simulink model "Modele_Principale"  (R2022b)
settings: Solver=ode3  StartTime=0.0  StopTime=150  FixedStep=0.05  RelTol=1e-3
model workspace (MAT data in the model file):
  D_Mesure = 0
values from neighbouring files (symbols this model uses):
  Acceleration_Max = 3.2    [Matlab_WorkSpace.mat]
  Distance_initial = 8    [Matlab_WorkSpace.mat]
  Frein_Max = -9    [Matlab_WorkSpace.mat]
  glissement = 0.22    [Matlab_WorkSpace.mat]
  r = 0.3    [Matlab_WorkSpace.mat]
  vehicule_half_length = 2.5    [Matlab_WorkSpace.mat]
libraries: sim3dautolib x2, slpidlib x2, sim3dprobsensorlib x1, sim3dlib x1
settings Model: Creator=Yoamiri  LastModifiedBy=Yoamiri
settings OptimizationCC: DefaultParameterBehavior=Inlined  EnhancedBackFolding=on  PassReuseOutputArgsAs=Individual arguments  ZeroExternalMemoryAtStartup=off  ZeroInternalMemoryAtStartup=off  OptimizeBlockOrder=speed  DifferentSizesBufferReuse=on  OptimizationCustomize=off  EfficientTunableParamExpr=on
settings DebuggingCC: ParameterTunabilityLossMsg=error
settings HardwareCC: ProdBitPerPointer=32  ProdBitPerSizeT=32  ProdBitPerPtrDiffT=32  ProdLargestAtomicFloat=None  ProdWordSize=32  ProdHWDeviceType=Atmel->AVR (32-bit)
settings SFSimCC: MATLABDynamicMemAlloc=off
settings RTWCC: Description=Embedded Coder  SystemTargetFile=ert.tlc  TemplateMakefile=ert_default_tmf  PortableWordSizes=on  CreateSILPILBlock=SIL
settings CodeAppCC: ForceParamTrailComments=on  IgnoreCustomStorageClasses=off  OperatorAnnotations=on  SimulinkDataObjDesc=on  SFDataObjDesc=on  InsertBlockDesc=on
settings ERTTargetCC: TargetLangStandard=C99 (ISO)  GenerateSampleERTMain=on  SupportVariableSizeSignals=on  InlinedParameterPlacement=NonHierarchical  ERTCustomFileTemplate=example_file_process.tlc

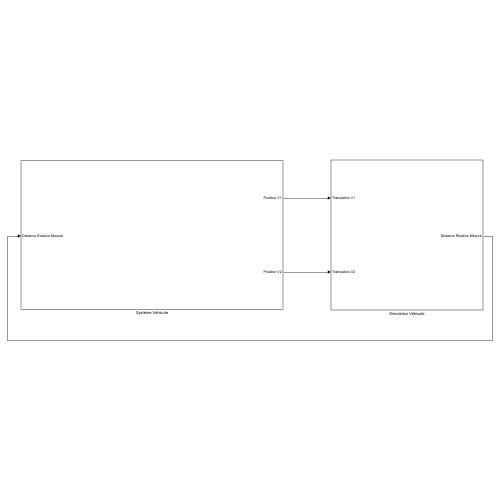
[thumbnail: Simulink's stored preview of the top-level diagram]
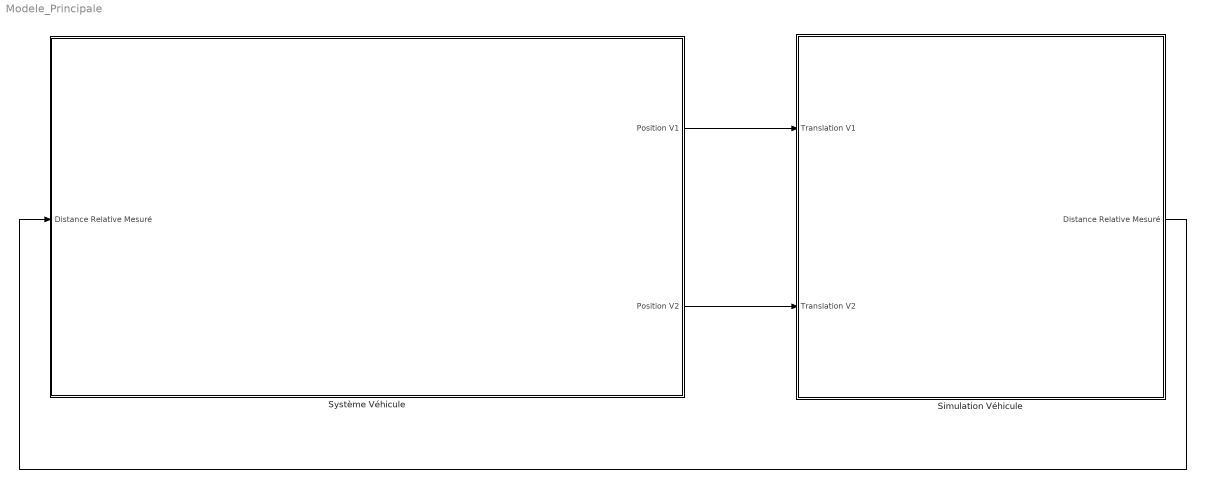
== system Modele_Principale ==
  Simulation Véhicule : Subsystem
  Système Véhicule : Subsystem
  wires:
  Système Véhicule/1(Position V1) -> Simulation Véhicule/1(Translation V1)
  Système Véhicule/2(Position V2) -> Simulation Véhicule/2(Translation V2)
  Simulation Véhicule/1(Distance Relative Mesuré) -> Système Véhicule/1(Distance Relative Mesuré)

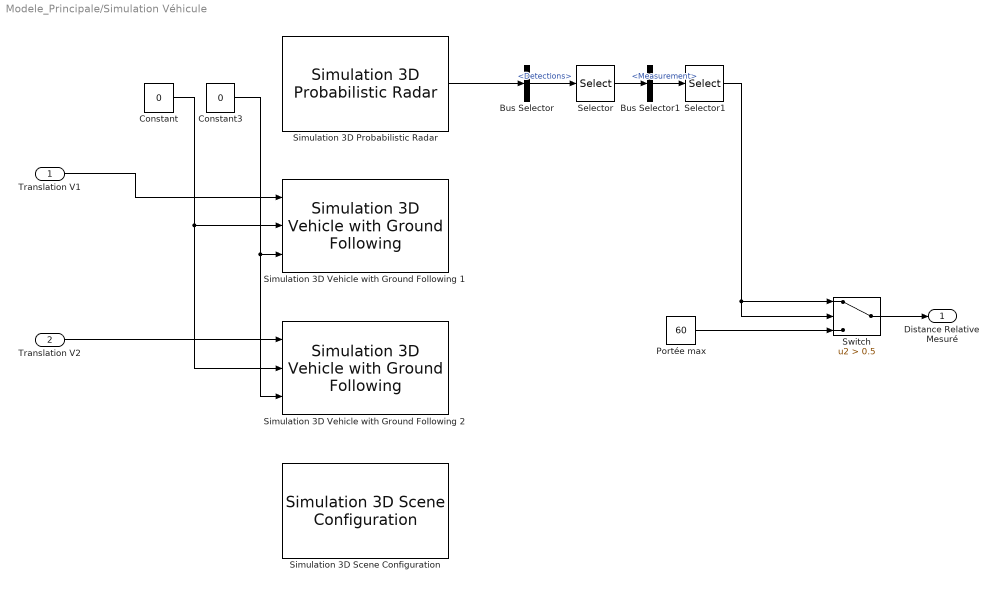
== system Modele_Principale/Simulation Véhicule ==
  Translation V1 : Inport
  Translation V2 : Inport  Port=2
  Bus Selector : BusSelector  OutputSignals=Detections
  Bus Selector1 : BusSelector  OutputSignals=Measurement
  Constant : Constant  Value=0
  Constant3 : Constant  Value=0
  Portée max : Constant  Value=60
  Selector : Selector  InputPortWidth=50  IndexOptions=Index vector (dialog)  Indices=[1]  OutputSizes=1
  Selector1 : Selector  InputPortWidth=6  IndexOptions=Index vector (dialog)  Indices=[1]  OutputSizes=1
  Simulation 3D Probabilistic Radar : sim3dprobsensorlib/Simulation 3D Probabilistic Radar  Priority=1  sensorTag=Sim3dSensor1  sensorId=1  sensorName=Sim3dSensor1  vehTagList={'Scene Origin';'Vehicule_Leader';'Vehicule_Suiveur'}  vehTag=Vehicule_Suiveur  mountLoc=Front bumper  offsetFlag=off  tmountOffset=[2.42, 0, 0.6]  rmountOffset=[0, 0, 0]  AzimuthResolution=4  ElevationResolution=10  RangeResolution=2.5  RangeRateResolution=0.5  AzimuthBiasFraction=0.1  ElevationBiasFraction=0.1  RangeBiasFraction=0.05  RangeRateBiasFraction=0.05  FieldOfView=[ 50, 10 ]  DetectionRange=[ 0.5, 200 ]  RangeRateLimits=[ -100, 100 ]  DetectionProbability=0.95  FalseAlarmRate=1e-6  ReferenceRange=180  ReferenceRCS=-10  HasElevation=on  HasRangeRate=on  HasNoise=on  HasFalseAlarms=on  InitialSeedSource=Repeatable  InitialSeed=0  MaxNumDetections=50  DetectionCoordinates=Ego Cartesian  SpecifyOutputBusName=off  BusName=BusSimulation3DRadarTruthSensor  SampleTime=-1  mountPoint=[2.42400002479553 0 0.5]  mountOrientation=[0 0 0]  aMode=3  ID=1
      settings: LibrarySourceBlock=drivingsim3d/Simulation 3D Probabilistic Radar
  Simulation 3D Scene Configuration : sim3dlib/Simulation 3D Scene Configuration  Priority=0  ProjectFormat=Default Scenes  SceneDesc=Straight road  ProjectName=C:\Program Files\MATLAB\R2022b\toolbox\shared\sim3d_projects\automotive_project\UE4\WindowsNoEditor\VehicleSimulation.exe  ScenePath=/Game/Maps/HwStrght  EnableOpenDRIVE=off  vehTagList={'Scene Origin';'Vehicule_Leader';'Vehicule_Suiveur'}  vehTag=Vehicule_Suiveur  OpVisEn=off  Ts=1/20  EnableWindow=on  EnableRemoteAccess=off  EnableWeather=off  SunAltitude=40.0  SunAzimuth=90  clouds=10  wind=1  fog=0  rain=0  EnableGeospatial=off  OriginHeight=200  OriginLatitude=40.744652  OriginLongitude=-73.988864  MapStyle=Aerial  AdditionalAssetIDs=[]  UseAdvancedSunSky=off  SolarTime=11  TimeZone=-5  Day=21  Month=9  Year=2022  UseDaylightSavingTime=on  DSTStartDay=10  DSTStartMonth=3  DSTEndDay=3  DSTEndMonth=11  DSTSwitchHour=2  sensorTag=MainCamera1  sensorId=1  sensorName=MainCamera1  mountLoc=Origin  offsetFlag=off  tmountOffset=[0, 0, 0]  rmountOffset=[0, 0, 0]  HorizontalResolution=1280  VerticalResolution=720  HorizontalFOV=60  mountPoint=[0 0 0]  mountOrientation=[0 0 0]  aMode=3  ID=1  GeoTrigger=Inactive
      settings: LibrarySourceBlock=drivingsim3d/Simulation 3D Scene Configuration
  Simulation 3D Vehicle with Ground Following 1 : sim3dautolib/Simulation 3D Vehicle with Ground Following  Priority=-1  PassVehMesh=Sedan  MeshPath=/MathWorksAutomotiveContent/Vehicles/Muscle/Meshes/SK_MuscleCar.SK_MuscleCar  TrackWidth=1.9  WheelBase=3  WheelRadius=0.35  VehColor=Blue  InitialPos=[0, 0, 0]  InitialRot=[0, 0, 0]  ActorName=Vehicule_Suiveur  SampleTime=-1  ActorType=SimulinkVehicle  ID=C  aMode=3  ActorTag=Vehicule_Suiveur  CoordinateScheme=ISO  VehLightsControl=off  HeadlightColor=[ 1, 1, 1 ]  HighBeamIntensity=100000  LowBeamIntensity=60000  HighBeamConeAngle=70  LowBeamConeAngle=70  LeftHeadlightOrientation=[ 0, 0 ]  RightHeadlightOrientation=[ 0, 0 ]  BrakelightIntensity=500  ReverselightIntensity=500  SignallightIntensity=500  SignallightPeriod=1  SignalPulseWidth=50  TransformOutportEnabled=off
      settings: LibrarySourceBlock=drivingsim3d/Simulation 3D Vehicle with Ground Following
  Simulation 3D Vehicle with Ground Following 2 : sim3dautolib/Simulation 3D Vehicle with Ground Following  Priority=-1  PassVehMesh=Sedan  MeshPath=/MathWorksAutomotiveContent/Vehicles/Muscle/Meshes/SK_MuscleCar.SK_MuscleCar  TrackWidth=1.9  WheelBase=3  WheelRadius=0.35  VehColor=White  InitialPos=[0, 0, 0]  InitialRot=[0, 0, 0]  ActorName=Vehicule_Leader  SampleTime=-1  ActorType=SimulinkVehicle  ID=C  aMode=3  ActorTag=Vehicule_Leader  CoordinateScheme=ISO  VehLightsControl=off  HeadlightColor=[ 1, 1, 1 ]  HighBeamIntensity=100000  LowBeamIntensity=60000  HighBeamConeAngle=70  LowBeamConeAngle=70  LeftHeadlightOrientation=[ 0, 0 ]  RightHeadlightOrientation=[ 0, 0 ]  BrakelightIntensity=500  ReverselightIntensity=500  SignallightIntensity=500  SignallightPeriod=1  SignalPulseWidth=50  TransformOutportEnabled=off
      settings: LibrarySourceBlock=drivingsim3d/Simulation 3D Vehicle with Ground Following
  Switch : Switch  Criteria=u2 > Threshold  Threshold=0.5  SaturateOnIntegerOverflow=off  InputSameDT=off
  Distance Relative Mesuré : Outport
  wires:
  Constant/1 -> Simulation 3D Vehicle with Ground Following 1/2, Simulation 3D Vehicle with Ground Following 2/2
  Constant3/1 -> Simulation 3D Vehicle with Ground Following 2/3, Simulation 3D Vehicle with Ground Following 1/3
  Simulation 3D Probabilistic Radar/1 -> Bus Selector/1
  Bus Selector/1 -> Selector/1  "<Detections>"
  Selector/1 -> Bus Selector1/1
  Bus Selector1/1 -> Selector1/1  "<Measurement>"
  Translation V2/1 -> Simulation 3D Vehicle with Ground Following 2/1
  Translation V1/1 -> Simulation 3D Vehicle with Ground Following 1/1
  Switch/1 -> Distance Relative Mesuré/1
  Selector1/1 -> Switch/1, Switch/2
  Portée max/1 -> Switch/3

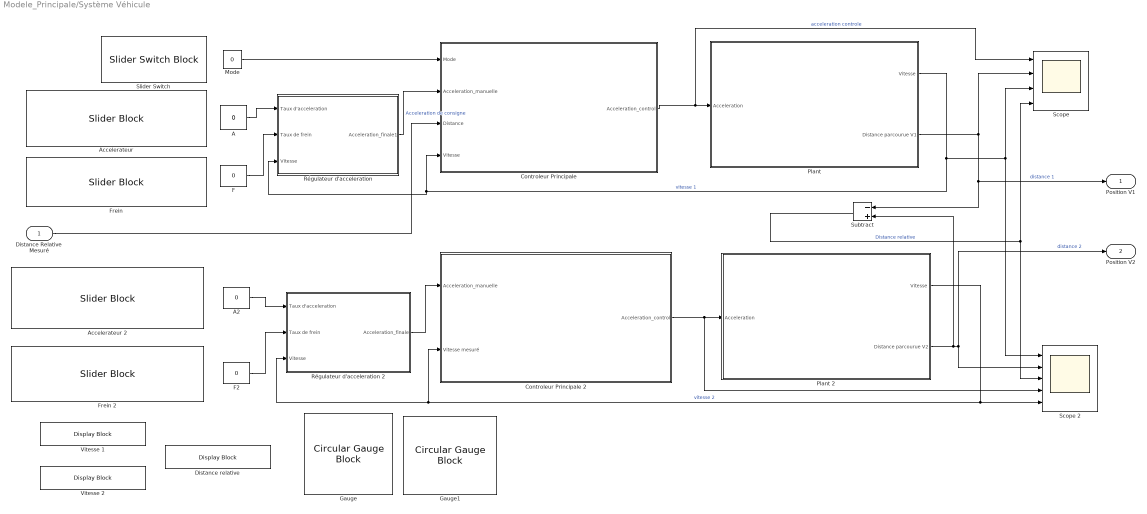
== system Modele_Principale/Système Véhicule ==
  Distance Relative Mesuré : Inport
  A : Constant  Value=0
  A2 : Constant  Value=0
  Accelerateur : SliderBlock  TickInterval=10
  Accelerateur 2 : SliderBlock  TickInterval=10
  Controleur Principale : Subsystem  TreatAsAtomicUnit=on
  Controleur Principale 2 : Subsystem
  Distance relative : DisplayBlock  LabelPosition=Hide  Transparency=1
  F : Constant  Value=0
  F2 : Constant  Value=0
  Frein : SliderBlock  TickInterval=10
  Frein 2 : SliderBlock  TickInterval=10
  Gauge : CircularGaugeBlock  ScaleMax=120
  Gauge1 : CircularGaugeBlock  ScaleMax=120
  Mode : Constant  Value=0  OutDataTypeStr=boolean
  Plant : Subsystem
  Plant 2 : Subsystem
  Régulateur d'acceleration : Subsystem
  Régulateur d'acceleration 2 : Subsystem
  Scope : Scope  NumInputPorts=4
  Scope 2 : Scope  NumInputPorts=5
  Slider Switch : SliderSwitchBlock
      settings: Values={{'Manuel', 'Auto'}, [1 0]}
  Subtract : Sum  Inputs=-+
  Vitesse 1 : DisplayBlock  LabelPosition=Hide  Transparency=1
  Vitesse 2 : DisplayBlock  LabelPosition=Hide  Transparency=1
  Position V1 : Outport
  Position V2 : Outport  Port=2
  wires:
  Controleur Principale 2/1(Acceleration_control) -> Plant 2/1(Acceleration), Scope 2/4
  A2/1 -> Régulateur d'acceleration 2/1(Taux d'acceleration)
  Régulateur d'acceleration 2/1(Acceleration_finale) -> Controleur Principale 2/1(Acceleration_manuelle)
  Régulateur d'acceleration/1(Acceleration_finale1) -> Controleur Principale/2(Acceleration_manuelle)  "Acceleration de consigne"
  Controleur Principale/1(Acceleration_control) -> Scope/1, Plant/1(Acceleration)  "acceleration controle"
  F2/1 -> Régulateur d'acceleration 2/2(Taux de frein)
  Plant/1(Vitesse) -> Scope/3, Scope 2/1, Régulateur d'acceleration/3(Vitesse), Controleur Principale/4(Vitesse)  "vitesse 1"
  Mode/1 -> Controleur Principale/1(Mode)
  Subtract/1 -> Scope/4, Scope 2/3  "Distance relative"
  Plant 2/1(Vitesse) -> Régulateur d'acceleration 2/3(Vitesse), Controleur Principale 2/2(Vitesse mesuré), Scope 2/5  "vitesse 2"
  Plant/2(Distance parcourue V1) -> Position V1/1, Subtract/1, Scope/2  "distance 1"
  Plant 2/2(Distance parcourue V2) -> Scope 2/2, Position V2/1, Subtract/2  "distance 2"
  A/1 -> Régulateur d'acceleration/1(Taux d'acceleration)
  F/1 -> Régulateur d'acceleration/2(Taux de frein)
  Distance Relative Mesuré/1 -> Controleur Principale/3(Distance)

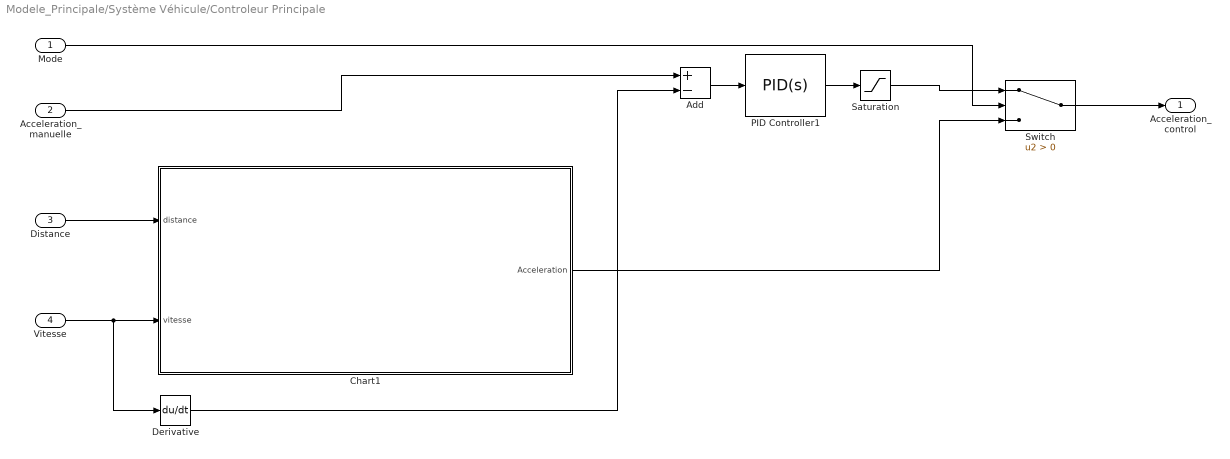
== system Modele_Principale/Système Véhicule/Controleur Principale ==
  Mode : Inport
  Acceleration_manuelle : Inport  Port=2
  Distance : Inport  Port=3
  Vitesse : Inport  Port=4
  Add : Sum  Inputs=+-
  Chart1 : Stateflow chart  TreatAsAtomicUnit=on
      settings: PortSchema="{\"entries\":[{\"content\":{\"sides\":[{\"content\":{\"connectorIds\":[\"In2\",\"In1\"]},\"type\":\"ConnectorPlacement.EquallySpacedRectSide\",\"uuid\":\"817b4df0-cad5-487b-96cc-92627ec0950c\"},{\"content\":{\"connectorIds\":[\"Out1\"],\"side\":\"RIGHT\"},\"type\":\"ConnectorPlacement.EquallySpacedRectSide\",\"uuid\":\"3ed398d5-bd25-476a-bdb3-4a370c0a56e0\"},{\"content\":{\"connectorIds\":[],\"side\":\"TOP\"},\"type\":\"ConnectorPlacement.EquallySpacedRectSide\",\"uuid\":\"2720e91f-838e-45a9-a5c0-db36849d5af3\"}]},\"type\":\"ConnectorPlacement.EquallySpacedConnector\",\"uuid\":\"053b983b-d27d-4c27-a764-ee3a54f47404\"}],\"packageUris\":[\"http://schema.mathworks.com/mf0/Connector/R2020b\"],\"version\":\"1.0\"}"
  Derivative : Derivative
  PID Controller1 : slpidlib/PID Controller  Controller=PID  Form=Parallel  TimeDomain=Continuous-time  UseExternalTs=off  SampleTime=-1  IntegratorMethod=Forward Euler  FilterMethod=Forward Euler  ControllerParametersSource=internal  P=4  I=1.5  UseKiTs=off  D=0  N=100  UseFilter=on  TunerSelectOption=Transfer Function Based (PID Tuner App)  InitialConditionSource=internal  InitialConditionForIntegrator=0  InitialConditionForFilter=0  DifferentiatorICPrevScaledInput=0  ExternalReset=none  TrackingMode=off  Kt=1  LimitOutput=off  SatLimitsSource=internal  UpperSaturationLimit=inf  LowerSaturationLimit=-inf  LinearizeAsGain=on  AntiWindupMode=none  Kb=1  LimitIntegrator=off  UpperIntegratorSaturationLimit=inf  LowerIntegratorSaturationLimit=-inf  POutMin=[]  POutMax=[]  IOutMin=[]  IOutMax=[]  DOutMin=[]  DOutMax=[]  NOutMin=[]  NOutMax=[]  SumOutMin=[]  SumOutMax=[]  SaturationOutMin=[]  SaturationOutMax=[]  PParamMin=[]  PParamMax=[]  IParamMin=[]  IParamMax=[]  DParamMin=[]  DParamMax=[]  NParamMin=[]  NParamMax=[]  KbParamMin=[]  KbParamMax=[]  KtParamMin=[]  KtParamMax=[]  KbOutMin=[]  KbOutMax=[]  KtOutMin=[]  KtOutMax=[]  IntegratorOutMin=[]  IntegratorOutMax=[]  FilterOutMin=[]  FilterOutMax=[]  SumI1OutMin=[]  SumI1OutMax=[]  SumI2OutMin=[]  SumI2OutMax=[]  SumI3OutMin=[]  SumI3OutMax=[]  SumI4OutMin=[]  SumI4OutMax=[]  SumDOutMin=[]  SumDOutMax=[]  DifferentiatorOutMin=[]  DifferentiatorOutMax=[]  FilterDiffOutCoefMin=[]  FilterDiffOutCoefMax=[]  ReciprocalOutMin=[]  ReciprocalOutMax=[]  SumDenOutMin=[]  SumDenOutMax=[]  SumNumOutMin=[]  SumNumOutMax=[]  DivideOutMin=[]  DivideOutMax=[]  UdiffTsProdOutMin=[]  UdiffTsProdOutMax=[]  NTsProdOutMin=[]  NTsProdOutMax=[]  UintegralTsProdOutMin=[]  UintegralTsProdOutMax=[]  UngainTsProdOutMin=[]  UngainTsProdOutMax=[]  ClampingZeroOutDataTypeStr=Inherit: Inherit via back propagation  ClampingZeroOutMin=[]  ClampingZeroOutMax=[]  FilterDenConstantOutDataTypeStr=Inherit: Inherit via back propagation  FilterDenConstantOutMin=[]  FilterDenConstantOutMax=[]  PCopyOutDataTypeStr=Inherit: Inherit via back propagation  PCopyOutMin=[]  PCopyOutMax=[]  NCopyOutDataTypeStr=Inherit: Inherit via back propagation  NCopyOutMin=[]  NCopyOutMax=[]  IntegratorContinuousStateAttributes=''  IntegratorStateMustResolveToSignalObject=off  IntegratorRTWStateStorageClass=Auto  FilterContinuousStateAttributes=''  FilterStateMustResolveToSignalObject=off  FilterRTWStateStorageClass=Auto  ParallelPVariant=InternalParameters  IdealPVariant=Disabled  IVariant=InternalParameters  DVariant=InternalParameters  IntegratorVariant=Continuous  SatVariant=Disabled  AWVariant=Passthrough  PCopyVariant=Disabled  TRVariant=Disabled  FdbkBlocksVariant=Forward  IdealPFdbkVariant=Disabled  SatFdbkVariant=Disabled  DerivativeFilterVariant=ContFilter  NVariant=InternalParameters  NCopyVariant=Disabled  FilterICVariant=InternalICsFilter  IntegratorICVariant=InternalICs  ExternalResetVariant=Disabled  TRSumVariant=Passthrough  SumFdbkVariant=Disabled  SumVariant=Sum_PID  TsampFilterVariant=InternalTs  TsampNgainVariant=Passthrough  TsampIntegralVariant=Passthrough  ExternalSaturationOutDataTypeStr=Inherit: Same as second input
  Saturation : Saturate  UpperLimit=Acceleration_Max  LowerLimit=Frein_Max  OutDataTypeStr=double
  Switch : Switch  Criteria=u2 > Threshold  OutDataTypeStr=double  SaturateOnIntegerOverflow=off  InputSameDT=off
  Acceleration_control : Outport
  wires:
  Add/1 -> PID Controller1/1
  PID Controller1/1 -> Saturation/1
  Chart1/1(Acceleration) -> Switch/3
  Saturation/1 -> Switch/1
  Distance/1 -> Chart1/2(distance)
  Mode/1 -> Switch/2
  Acceleration_manuelle/1 -> Add/1
  Switch/1 -> Acceleration_control/1
  Vitesse/1 -> Derivative/1, Chart1/1(vitesse)
  Derivative/1 -> Add/2

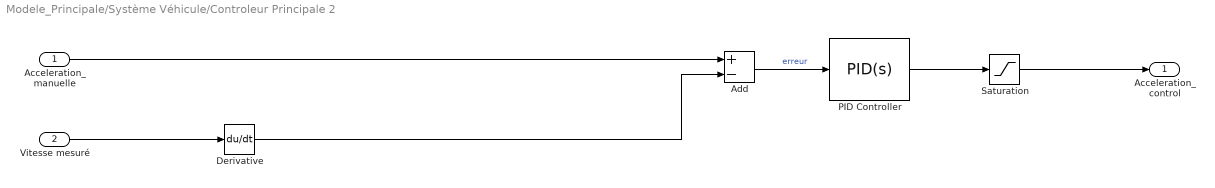
== system Modele_Principale/Système Véhicule/Controleur Principale 2 ==
  Acceleration_manuelle : Inport
  Vitesse mesuré : Inport  Port=2
  Add : Sum  Inputs=+-
  Derivative : Derivative
  PID Controller : slpidlib/PID Controller  Controller=PID  Form=Parallel  TimeDomain=Continuous-time  UseExternalTs=off  SampleTime=-1  IntegratorMethod=Forward Euler  FilterMethod=Forward Euler  ControllerParametersSource=internal  P=4  I=1.5  UseKiTs=off  D=0  N=100  UseFilter=on  TunerSelectOption=Transfer Function Based (PID Tuner App)  InitialConditionSource=internal  InitialConditionForIntegrator=0  InitialConditionForFilter=0  DifferentiatorICPrevScaledInput=0  ExternalReset=none  TrackingMode=off  Kt=1  LimitOutput=off  SatLimitsSource=internal  UpperSaturationLimit=inf  LowerSaturationLimit=-inf  LinearizeAsGain=on  AntiWindupMode=none  Kb=1  LimitIntegrator=off  UpperIntegratorSaturationLimit=inf  LowerIntegratorSaturationLimit=-inf  POutMin=[]  POutMax=[]  IOutMin=[]  IOutMax=[]  DOutMin=[]  DOutMax=[]  NOutMin=[]  NOutMax=[]  SumOutMin=[]  SumOutMax=[]  SaturationOutMin=[]  SaturationOutMax=[]  PParamMin=[]  PParamMax=[]  IParamMin=[]  IParamMax=[]  DParamMin=[]  DParamMax=[]  NParamMin=[]  NParamMax=[]  KbParamMin=[]  KbParamMax=[]  KtParamMin=[]  KtParamMax=[]  KbOutMin=[]  KbOutMax=[]  KtOutMin=[]  KtOutMax=[]  IntegratorOutMin=[]  IntegratorOutMax=[]  FilterOutMin=[]  FilterOutMax=[]  SumI1OutMin=[]  SumI1OutMax=[]  SumI2OutMin=[]  SumI2OutMax=[]  SumI3OutMin=[]  SumI3OutMax=[]  SumI4OutMin=[]  SumI4OutMax=[]  SumDOutMin=[]  SumDOutMax=[]  DifferentiatorOutMin=[]  DifferentiatorOutMax=[]  FilterDiffOutCoefMin=[]  FilterDiffOutCoefMax=[]  ReciprocalOutMin=[]  ReciprocalOutMax=[]  SumDenOutMin=[]  SumDenOutMax=[]  SumNumOutMin=[]  SumNumOutMax=[]  DivideOutMin=[]  DivideOutMax=[]  UdiffTsProdOutMin=[]  UdiffTsProdOutMax=[]  NTsProdOutMin=[]  NTsProdOutMax=[]  UintegralTsProdOutMin=[]  UintegralTsProdOutMax=[]  UngainTsProdOutMin=[]  UngainTsProdOutMax=[]  ClampingZeroOutDataTypeStr=Inherit: Inherit via back propagation  ClampingZeroOutMin=[]  ClampingZeroOutMax=[]  FilterDenConstantOutDataTypeStr=Inherit: Inherit via back propagation  FilterDenConstantOutMin=[]  FilterDenConstantOutMax=[]  PCopyOutDataTypeStr=Inherit: Inherit via back propagation  PCopyOutMin=[]  PCopyOutMax=[]  NCopyOutDataTypeStr=Inherit: Inherit via back propagation  NCopyOutMin=[]  NCopyOutMax=[]  IntegratorContinuousStateAttributes=''  IntegratorStateMustResolveToSignalObject=off  IntegratorRTWStateStorageClass=Auto  FilterContinuousStateAttributes=''  FilterStateMustResolveToSignalObject=off  FilterRTWStateStorageClass=Auto  ParallelPVariant=InternalParameters  IdealPVariant=Disabled  IVariant=InternalParameters  DVariant=InternalParameters  IntegratorVariant=Continuous  SatVariant=Disabled  AWVariant=Passthrough  PCopyVariant=Disabled  TRVariant=Disabled  FdbkBlocksVariant=Forward  IdealPFdbkVariant=Disabled  SatFdbkVariant=Disabled  DerivativeFilterVariant=ContFilter  NVariant=InternalParameters  NCopyVariant=Disabled  FilterICVariant=InternalICsFilter  IntegratorICVariant=InternalICs  ExternalResetVariant=Disabled  TRSumVariant=Passthrough  SumFdbkVariant=Disabled  SumVariant=Sum_PID  TsampFilterVariant=InternalTs  TsampNgainVariant=Passthrough  TsampIntegralVariant=Passthrough  ExternalSaturationOutDataTypeStr=Inherit: Same as second input
  Saturation : Saturate  UpperLimit=Acceleration_Max  LowerLimit=Frein_Max
  Acceleration_control : Outport
  wires:
  Vitesse mesuré/1 -> Derivative/1
  Derivative/1 -> Add/2
  Add/1 -> PID Controller/1  "erreur"
  PID Controller/1 -> Saturation/1
  Acceleration_manuelle/1 -> Add/1
  Saturation/1 -> Acceleration_control/1

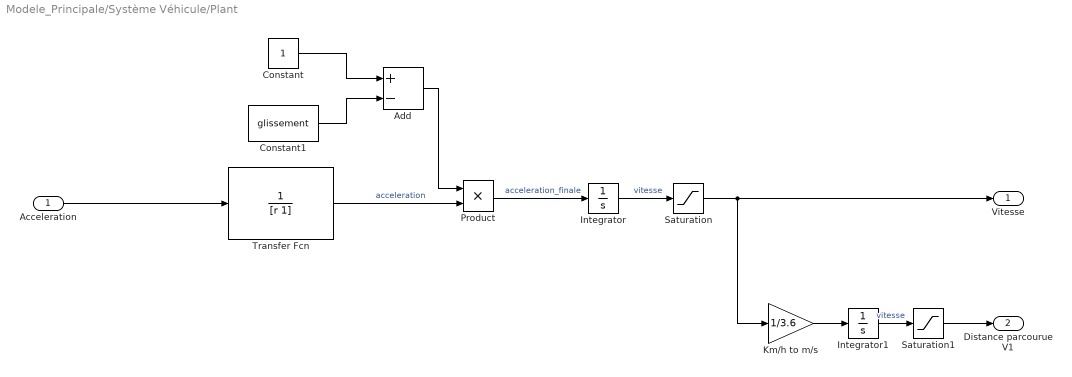
== system Modele_Principale/Système Véhicule/Plant ==
  Acceleration : Inport
  Add : Sum  Inputs=+-
  Constant : Constant
  Constant1 : Constant  Value=glissement
  Integrator : Integrator
  Integrator1 : Integrator
  Km/h to m/s : Gain  Gain=1/3.6
  Product : Product
  Saturation : Saturate  UpperLimit=120  LowerLimit=0
  Saturation1 : Saturate  UpperLimit=inf  LowerLimit=0
  Transfer Fcn : TransferFcn  Denominator=[r 1]
  Vitesse : Outport
  Distance parcourue V1 : Outport  Port=2
  wires:
  Acceleration/1 -> Transfer Fcn/1
  Product/1 -> Integrator/1  "acceleration_finale"
  Transfer Fcn/1 -> Product/2  "acceleration"
  Constant/1 -> Add/1
  Constant1/1 -> Add/2
  Add/1 -> Product/1
  Integrator1/1 -> Saturation1/1  "vitesse"
  Saturation/1 -> Vitesse/1, Km/h to m/s/1
  Saturation1/1 -> Distance parcourue V1/1
  Km/h to m/s/1 -> Integrator1/1
  Integrator/1 -> Saturation/1  "vitesse"

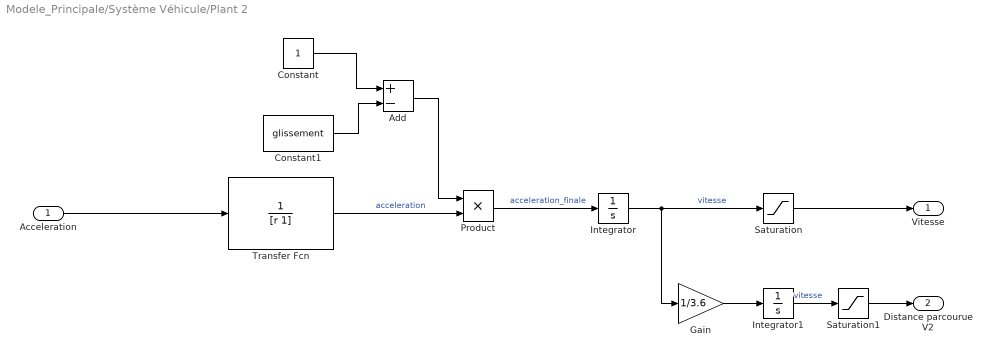
== system Modele_Principale/Système Véhicule/Plant 2 ==
  Acceleration : Inport
  Add : Sum  Inputs=+-
  Constant : Constant
  Constant1 : Constant  Value=glissement
  Gain : Gain  Gain=1/3.6
  Integrator : Integrator
  Integrator1 : Integrator  InitialCondition=Distance_initial+vehicule_half_length
  Product : Product
  Saturation : Saturate  UpperLimit=120  LowerLimit=0
  Saturation1 : Saturate  UpperLimit=inf  LowerLimit=0
  Transfer Fcn : TransferFcn  Denominator=[r 1]
  Vitesse : Outport
  Distance parcourue V2 : Outport  Port=2
  wires:
  Acceleration/1 -> Transfer Fcn/1
  Product/1 -> Integrator/1  "acceleration_finale"
  Transfer Fcn/1 -> Product/2  "acceleration"
  Constant/1 -> Add/1
  Constant1/1 -> Add/2
  Add/1 -> Product/1
  Integrator/1 -> Saturation/1, Gain/1  "vitesse"
  Integrator1/1 -> Saturation1/1  "vitesse"
  Gain/1 -> Integrator1/1
  Saturation/1 -> Vitesse/1
  Saturation1/1 -> Distance parcourue V2/1

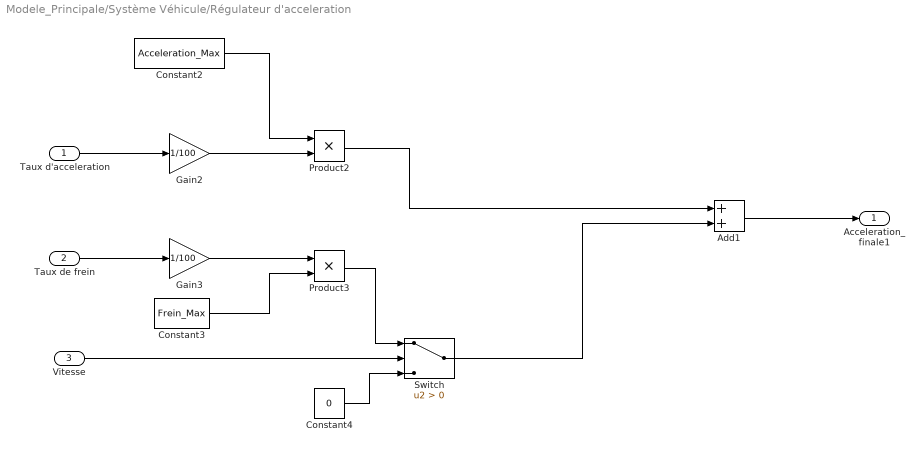
== system Modele_Principale/Système Véhicule/Régulateur d'acceleration ==
  Taux d'acceleration : Inport
  Taux de frein : Inport  Port=2
  Vitesse : Inport  Port=3
  Add1 : Sum
  Constant2 : Constant  Value=Acceleration_Max
  Constant3 : Constant  Value=Frein_Max
  Constant4 : Constant  Value=0
  Gain2 : Gain  Gain=1/100
  Gain3 : Gain  Gain=1/100
  Product2 : Product
  Product3 : Product
  Switch : Switch  Criteria=u2 > Threshold  SaturateOnIntegerOverflow=off  InputSameDT=off
  Acceleration_finale1 : Outport
  wires:
  Constant4/1 -> Switch/3
  Product3/1 -> Switch/1
  Vitesse/1 -> Switch/2
  Switch/1 -> Add1/2
  Product2/1 -> Add1/1
  Taux d'acceleration/1 -> Gain2/1
  Gain3/1 -> Product3/1
  Add1/1 -> Acceleration_finale1/1
  Constant2/1 -> Product2/1
  Taux de frein/1 -> Gain3/1
  Gain2/1 -> Product2/2
  Constant3/1 -> Product3/2

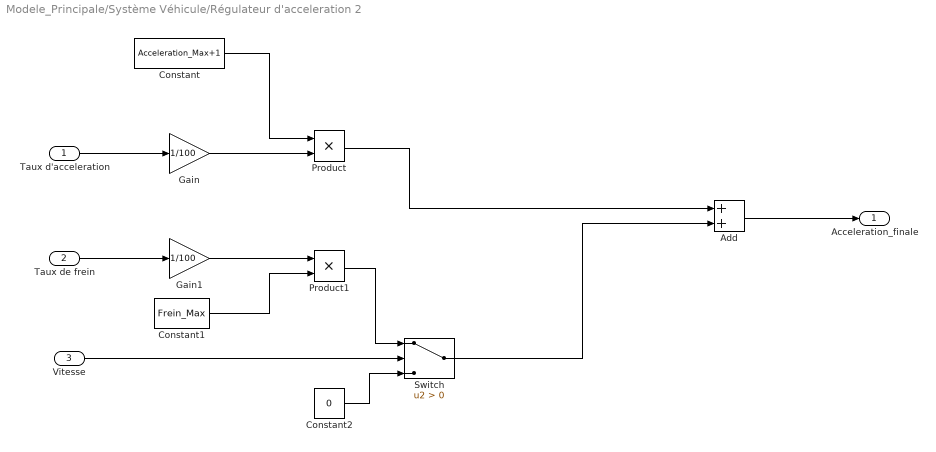
== system Modele_Principale/Système Véhicule/Régulateur d'acceleration 2 ==
  Taux d'acceleration : Inport
  Taux de frein : Inport  Port=2
  Vitesse : Inport  Port=3
  Add : Sum
  Constant : Constant  Value=Acceleration_Max+1
  Constant1 : Constant  Value=Frein_Max
  Constant2 : Constant  Value=0
  Gain : Gain  Gain=1/100
  Gain1 : Gain  Gain=1/100
  Product : Product
  Product1 : Product
  Switch : Switch  Criteria=u2 > Threshold  SaturateOnIntegerOverflow=off  InputSameDT=off
  Acceleration_finale : Outport
  wires:
  Taux de frein/1 -> Gain1/1
  Taux d'acceleration/1 -> Gain/1
  Constant1/1 -> Product1/2
  Constant/1 -> Product/1
  Gain/1 -> Product/2
  Gain1/1 -> Product1/1
  Product/1 -> Add/1
  Add/1 -> Acceleration_finale/1
  Vitesse/1 -> Switch/2
  Product1/1 -> Switch/1
  Switch/1 -> Add/2
  Constant2/1 -> Switch/3

== stateflow chart Modele_Principale/Système Véhicule/Controleur Principale/Chart1 ==
  state Stop
    entry:
    Acceleration = 0.0;
  state Frein_sec
    during:
    Frein_Max = -10;
    Acceleration = 0.95*Frein_Max;
  state En_file
    state Accelerer
      during:
      Acceleration = niveau_acceleration(distance);
    state Freiner
      during:
      Acceleration = niveau_frein(distance,vitesse);
    (default) -> Accelerer
    Freiner -> Accelerer [order 1] : [distance>=distance_securite(vitesse)]
    Accelerer -> Freiner : [distance<distance_securite(vitesse)]
  state En_route_libre
    during:
    Acceleration = accelerer_librement(vitesse);
  (default) -> Stop
  Stop -> En_file : [distance>=8]
  Freiner -> Stop [order 2] : [vitesse<=0.1]
  Frein_sec -> Stop [order 1] : [vitesse<=0.1]
  Frein_sec -> En_file [order 2] : [distance>5]
  En_file -> Frein_sec [order 1] : [distance<5 && vitesse>8]
  En_route_libre -> Freiner : [distance<distance_securite(vitesse)]
  En_file -> En_route_libre [order 2] : [distance>distance_securite(vitesse)]
  data: v function_input; d function_output; d function_input; a function_output; d function_input; a function_output; v function_input; v function_input; a function_output; Acceleration output; vitesse input; distance input; Frein_Max local
  function d = distance_securite(v):
    | function d = distance_securite(v)
    |     % v (Vitesse de vehicule en Km/h)
    |     % d (Distance parcourue en m)
    |     dmin = 8;
    |     Tbasse  = 0.9;
    |     Thaute  = 1.5;
    |     if(v>=5 && v<=100)
    | 
    |         d = dmin + (Tbasse * (v/3.6));
    |     elseif(v>90)
    |         d = dmin + (Thaute * (v/3.6));
    |     else
    |         d = dmin;
    |     end
    | 
    | end
  function a = niveau_acceleration(d):
    | function a = niveau_acceleration(d)
    | 
    |     Acceleration_Max = 3.8; %Acceleration en Km/h/s
    |     if(d<4.5)
    |         a = 0.05*Acceleration_Max;
    |     elseif(d>=4.5 && d<6)
    |         a = 0.2*Acceleration_Max;
    |     elseif(d>=6 && d<10)
    |         a = 0.3*Acceleration_Max;
    |     elseif(d>=10 && d<20)
    |         a = 0.55*Acceleration_Max;
    |     elseif(d>=20 && d<32)
    |         a = 0.8*Acceleration_Max;
    |     else
    |         a = 0.9*Acceleration_Max;
    |     end
    | end
  function a = niveau_frein(d,v):
    | function a = niveau_frein(d,v)
    | 
    |     Frein_Max = -9;
    |     if(v>0)
    |         if(d<8)
    |             if(v>=15)
    |                 a = 0.9*Frein_Max;
    |             elseif(v>=2 && v<15)
    |                 a = 0.7*Frein_Max;
    |             elseif(v>0 && v<2)
    |                 a = 0.48*Frein_Max;
    |             else
    |                 a = 0;
    |             end
    |         elseif(d>=8 && d<12)
    |             if(v>8)
    |                 a = 0.85*Frein_Max;
    |             else
    |                 a = 0.7*Frein_Max;
    |             end
    |         elseif(d>=12 && d<18)
    |             a = 0.5*Frein_Max;
    |         elseif(d>=18 && d<30)
    |             if(v>50)
    |                 a = 0.40*Frein_Max;
    |             else
    |                 a = 0.25*Frein_Max;
    |             end
    |         else
    |             if(v>90)
    |                 a = 0.25*Frein_Max;
    |             else
    |                 a = 0.10*Frein_Max;
    |             end
    |         end
    |     else
    |         a = 0;
    |     end
    | end
  function a = accelerer_librement(v):
    | function a = accelerer_librement(v)
    |     
    |     Vitesse_Max = 120;
    |     Acceleration_Max = 3.8;
    |     
    |     if(v<=Vitesse_Max)
    |         a = Acceleration_Max;
    |     else
    |         a = 0.0;
    |     end
    | end
